simulink model "MNIST_1level_NN"  (R2015b)
settings: Solver=VariableStepAuto  StartTime=0.0  StopTime=10.0  RelTol=1e-3
libraries: neural x7
(part 2 of 2)

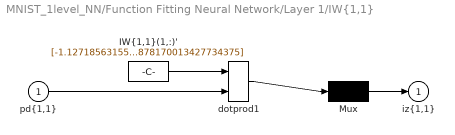
== system MNIST_1level_NN/Function Fitting Neural Network/Layer 1/IW{1,1} ==
  "pd{1,1}" : Inport  PortDimensions=717
      mask Display: e = 0.06;c1 = [120 230 180]/255;c2 = ([120 230 180]+0)/(256+128);c3 = ([120 230 180]+128)/(256+128);patch([0 1 1 0],[0 0 1 1],c1);patch([0 1 1 1-e 1-e 0+e],[0 0 1 1-e 0+e 0+e],c2);patch([0 0 1 1-e 0+e 0+e],[0 1 1 1-e 1-e 0+e],c3);plot([0 1 1 0 0],[0 0 1 1 0]);
  "IW{1,1}(1,:)'" : Constant  Value=[-1.1271856315593755670789732903358526527881622314453125;-1.1682507171942690948895915425964631140232086181640625;1.419847346731416326548469442059285938739776611328125;-1.36592089746078304557386218220926821231842041015625;-1.8771610426523874792792412335984408855438232421875;-0.455264915461362884574469944709562696516513824462890625;-1.1418628349723525250425382182584144175052642822265625;-1.136235914389979395622276570065878331661224365234375;-1.238786996007491314486514966120012104511260986328125;-1.2696468818339834427888490608893334865570068359375;1.73648660508436858407321778940968215465545654296875;-1.1712986247300849473873540773638524115085601806640625;-1.1050074866948644825015435344539582729339599609375;-1.1280337612593041018982376044732518494129180908203125;0.05620978092885971222347762932258774526417255401611328125;0.60097682395298590574128638763795606791973114013671875;-0.34543548989132977222737963529652915894985198974609375;-1.2533656709485720970320699052535928785800933837890625;1.349426984114299177264229001593776047229766845703125;-1.0955243382273101016011196406907401978969573974609375;1.26920278990640067462436491041444242000579833984375;1.8974440736891897696381192872649990022182464599609375;-0.867211887137548043114065876579843461513519287109375;0.441412329569272621210274110126192681491374969482421875;-1.1706813346600186687140876529156230390071868896484375;-1.177574319183268602984071549144573509693145751953125;-0.19702421990876028967676347747328691184520721435546875;-0.01191338623542848029757124095340259373188018798828125;0.0380604819739614741447297774357139132916927337646484375;0.86233452856553827192698236103751696646213531494140625;-1.739353512949751934257847096887417137622833251953125;-1.453773759185859493214820759021677076816558837890625;0.242249218246049002889463963583693839609622955322265625;-0.418613134782295670532903386629186570644378662109375;-0.179629427862431134688137035482213832437992095947265625;0.28210425444926823246305502834729850292205810546875;-1.6028676494376998817870116909034550189971923828125;0.2461683377036456843445222375521552748978137969970703125;0.707794344515888074198528556735254824161529541015625;0.30169678570108171555830267607234418392181396484375;0.7349710559525330921815111651085317134857177734375;-0.50331675576628309709548148020985536277294158935546875;0.96702088088355175887755876829032786190509796142578125;-0.43092743646723763450978594846674241125583648681640625;0.610089152153423963653722239541821181774139404296875;0.1633501147850167367625573433542740531265735626220703125;-0.449832971966681094411200092508806847035884857177734375;0.287603025350721741570936274001724086701869964599609375;-0.1369371527832669854785052621082286350429058074951171875;0.19556450742950826082733328803442418575286865234375;-0.0339328055533630601470207466263673268258571624755859375;0.1503621412636688692288089441717602312564849853515625;-0.1248641326846597066069222137230099178850650787353515625;0.113543479471111596890153805361478589475154876708984375;-0.62161111798026158492547210698830895125865936279296875;-0.27122282363050753684063920445623807609081268310546875;-0.45303470725305938771043656743131577968597412109375;0.14966949002307827765179126799921505153179168701171875;0.38088039712648547041595747941755689680576324462890625;-0.13199812501637797623743608710356056690216064453125;-0.167123462412796353060429055403801612555980682373046875;0.047867311970589500325079512776937917806208133697509765625;-0.11314410768925330097456338762640370987355709075927734375;0.02173742792166623305494255191661068238317966461181640625;-0.06886941982662098116207971543190069496631622314453125;0.1781361093339991763517815570594393648207187652587890625;-0.348689216665033552278174511229735799133777618408203125;0.092342387746760457023498247508541680872440338134765625;0.0923960665686115178996118402210413478314876556396484375;0.042442367801985493580563257864923798479139804840087890625;0.11181813532557392798505446762646897695958614349365234375 ...(+38193 chars)]
      mask Display: e = 0.06;c1 = [120 150 230]/255;c2 = ([120 150 230]+0)/383;c3 = ([120 150 230]+128)/383;patch([0 1 1 0],[0 0 1 1],c1);patch([0 1 1 1-e 1-e 0+e],[0 0 1 1-e 0+e 0+e],c2);patch([0 0 1 1-e 0+e 0+e],[0 1 1 1-e 1-e 0+e],c3);plot([0 1 1 0 0],[0 0 1 1 0]);disp('Weights');
  Mux : Mux  Inputs=1
      mask Display: e = 0.06;c1 = [120 150 230]/255;c2 = ([120 150 230]+0)/383;c3 = ([120 150 230]+128)/383;patch([0 1 1 0],[0 0 1 1],c1);patch([0 1 1 1-e 1-e 0+e],[0 0 1 1-e 0+e 0+e],c2);patch([0 0 1 1-e 0+e 0+e],[0 1 1 1-e 1-e 0+e],c3);plot([0 1 1 0 0],[0 0 1 1 0]);disp('Mux');
  dotprod1 : neural/Weight Functions/dotprod
  "iz{1,1}" : Outport
      mask Display: e = 0.06;c1 = [120 230 180]/255;c2 = ([120 230 180]+0)/(256+128);c3 = ([120 230 180]+128)/(256+128);patch([0 1 1 0],[0 0 1 1],c1);patch([0 1 1 1-e 1-e 0+e],[0 0 1 1-e 0+e 0+e],c2);patch([0 0 1 1-e 0+e 0+e],[0 1 1 1-e 1-e 0+e],c3);plot([0 1 1 0 0],[0 0 1 1 0]);
  wires:
  "IW{1,1}(1,:)'"/1 -> dotprod1/1
  "pd{1,1}"/1 -> dotprod1/2
  dotprod1/1 -> Mux/1
  Mux/1 -> "iz{1,1}"/1

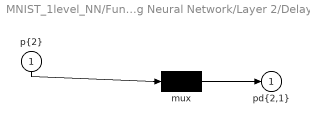
== system MNIST_1level_NN/Function Fitting Neural Network/Layer 2/Delays 1 ==
  "p{2}" : Inport  PortDimensions=1
      mask Display: e = 0.06;c1 = [120 230 180]/255;c2 = ([120 230 180]+0)/(256+128);c3 = ([120 230 180]+128)/(256+128);patch([0 1 1 0],[0 0 1 1],c1);patch([0 1 1 1-e 1-e 0+e],[0 0 1 1-e 0+e 0+e],c2);patch([0 0 1 1-e 0+e 0+e],[0 1 1 1-e 1-e 0+e],c3);plot([0 1 1 0 0],[0 0 1 1 0]);
  mux : Mux  Inputs=1
      mask Display: e = 0.06;c1 = [120 150 230]/255;c2 = ([120 150 230]+0)/383;c3 = ([120 150 230]+128)/383;patch([0 1 1 0],[0 0 1 1],c1);patch([0 1 1 1-e 1-e 0+e],[0 0 1 1-e 0+e 0+e],c2);patch([0 0 1 1-e 0+e 0+e],[0 1 1 1-e 1-e 0+e],c3);plot([0 1 1 0 0],[0 0 1 1 0]);disp('Mux')
  "pd{2,1}" : Outport
      mask Display: e = 0.06;c1 = [120 230 180]/255;c2 = ([120 230 180]+0)/(256+128);c3 = ([120 230 180]+128)/(256+128);patch([0 1 1 0],[0 0 1 1],c1);patch([0 1 1 1-e 1-e 0+e],[0 0 1 1-e 0+e 0+e],c2);patch([0 0 1 1-e 0+e 0+e],[0 1 1 1-e 1-e 0+e],c3);plot([0 1 1 0 0],[0 0 1 1 0]);
  wires:
  "p{2}"/1 -> mux/1
  mux/1 -> "pd{2,1}"/1

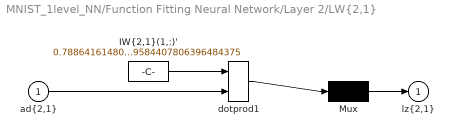
== system MNIST_1level_NN/Function Fitting Neural Network/Layer 2/LW{2,1} ==
  "ad{2,1}" : Inport  PortDimensions=1
      mask Display: e = 0.06;c1 = [120 230 180]/255;c2 = ([120 230 180]+0)/(256+128);c3 = ([120 230 180]+128)/(256+128);patch([0 1 1 0],[0 0 1 1],c1);patch([0 1 1 1-e 1-e 0+e],[0 0 1 1-e 0+e 0+e],c2);patch([0 0 1 1-e 0+e 0+e],[0 1 1 1-e 1-e 0+e],c3);plot([0 1 1 0 0],[0 0 1 1 0]);
  "IW{2,1}(1,:)'" : Constant  Value=0.7886416148075612309042980996309779584407806396484375
      mask Display: e = 0.06;c1 = [120 150 230]/255;c2 = ([120 150 230]+0)/383;c3 = ([120 150 230]+128)/383;patch([0 1 1 0],[0 0 1 1],c1);patch([0 1 1 1-e 1-e 0+e],[0 0 1 1-e 0+e 0+e],c2);patch([0 0 1 1-e 0+e 0+e],[0 1 1 1-e 1-e 0+e],c3);plot([0 1 1 0 0],[0 0 1 1 0]);disp('weights');
  Mux : Mux  Inputs=1
      mask Display: e = 0.06;c1 = [120 150 230]/255;c2 = ([120 150 230]+0)/383;c3 = ([120 150 230]+128)/383;patch([0 1 1 0],[0 0 1 1],c1);patch([0 1 1 1-e 1-e 0+e],[0 0 1 1-e 0+e 0+e],c2);patch([0 0 1 1-e 0+e 0+e],[0 1 1 1-e 1-e 0+e],c3);plot([0 1 1 0 0],[0 0 1 1 0]);disp('Mux');
  dotprod1 : neural/Weight Functions/dotprod
  "lz{2,1}" : Outport
      mask Display: e = 0.06;c1 = [120 230 180]/255;c2 = ([120 230 180]+0)/(256+128);c3 = ([120 230 180]+128)/(256+128);patch([0 1 1 0],[0 0 1 1],c1);patch([0 1 1 1-e 1-e 0+e],[0 0 1 1-e 0+e 0+e],c2);patch([0 0 1 1-e 0+e 0+e],[0 1 1 1-e 1-e 0+e],c3);plot([0 1 1 0 0],[0 0 1 1 0]);
  wires:
  "IW{2,1}(1,:)'"/1 -> dotprod1/1
  "ad{2,1}"/1 -> dotprod1/2
  dotprod1/1 -> Mux/1
  Mux/1 -> "lz{2,1}"/1
